simulink model "fault_tolerant_controller"  (R2015a)
settings: Solver=ode45  SolverMode=SingleTasking  StartTime=0.0  StopTime=150  RelTol=1e-3
values from neighbouring files (symbols this model uses):
  g = 9.8    [model.mat]
  Kd = 1e-06    [model.mat]
  Kt = 1    [model.mat]
  U0 = 120    [model.mat]
  X0 = 0    [model.mat]
  Y0 = 5000    [model.mat]
undefined symbols (not defined in the file or in its folder): magnitude
libraries: simulink x53, aerolibatmos2 x12, aerolibconvert2 x4
(part 1 of 2)
settings Model: CovMetricSettings=dwe  CovHtmlReporting=off  covSaveCumulativeToWorkspaceVar=off  CovSaveSingleToWorkspaceVar=off  CovExternalEMLEnable=on  Creator=jomig  LastModifiedBy=Tiago Alexandre
settings DataIOCC: LimitDataPoints=off  SaveFormat=Dataset
settings DebuggingCC: SFUnexpectedBacktrackingDiag=error  SFNoUnconditionalDefaultTransitionDiag=error
settings HardwareCC: ProdBitPerPointer=64  ProdLargestAtomicFloat=Float  ProdIntDivRoundTo=Zero  ProdEndianess=LittleEndian  ProdHWDeviceType=Specified
settings ModelReferenceCC: PropagateSignalLabelsOutOfModel=on
settings GRTTargetCC: TargetLangStandard=C99 (ISO)  GeneratePreprocessorConditionals=Use local settings

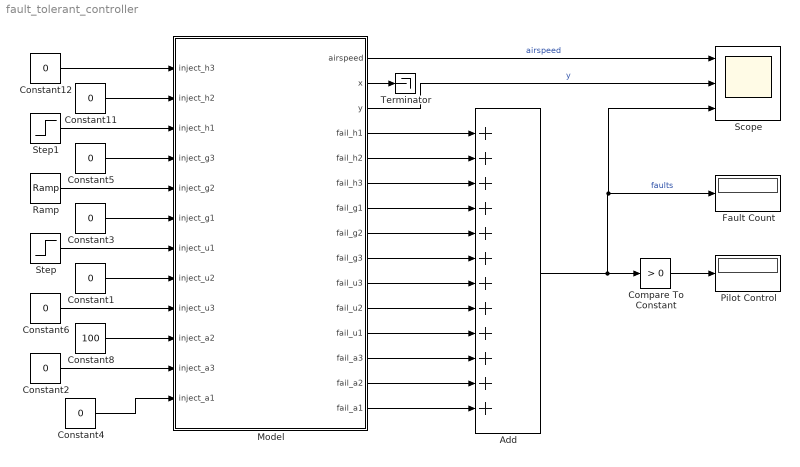
== system fault_tolerant_controller ==
  Add : Sum  Inputs=++++++++++++
  Compare To Constant : simulink/Logic and Bit Operations/Compare To Constant  relop=>  const=0  OutDataTypeStr=boolean
  Constant{1..6,11..12} (8 alike) : Constant  Value=0
  Constant8 : Constant  Value=100
  Fault Count : Display
  Model : Subsystem
  Pilot Control : Display
  Ramp : simulink/Sources/Ramp  slope=5  start=50  X0=0
  Scope : Scope  NumInputPorts=3
      settings: TimeRange=150  YMin=119~4800~1  YMax=121~5600~4
  Step : Step  Time=25  After=25  SampleTime=0
  Step1 : Step  Time=35  After=-5000  SampleTime=0
  Terminator : Terminator
  wires:
  Model/1(airspeed) -> Scope/1  "airspeed"
  Model/4(fail_h1) -> Add/1
  Model/5(fail_h2) -> Add/2
  Model/6(fail_h3) -> Add/3
  Model/7(fail_g1) -> Add/4
  Model/8(fail_g2) -> Add/5
  Model/9(fail_g3) -> Add/6
  Model/10(fail_u3) -> Add/7
  Model/11(fail_u2) -> Add/8
  Model/12(fail_u1) -> Add/9
  Model/13(fail_a3) -> Add/10
  Model/14(fail_a2) -> Add/11
  Model/15(fail_a1) -> Add/12
  Compare To Constant/1 -> Pilot Control/1
  Add/1 -> Scope/3, Fault Count/1, Compare To Constant/1  "faults"
  Constant8/1 -> Model/10(inject_a2)
  Constant6/1 -> Model/9(inject_u3)
  Constant1/1 -> Model/8(inject_u2)
  Step/1 -> Model/7(inject_u1)
  Constant3/1 -> Model/6(inject_g1)
  Ramp/1 -> Model/5(inject_g2)
  Constant5/1 -> Model/4("inject_g3 ")
  Step1/1 -> Model/3(inject_h1)
  Constant11/1 -> Model/2(inject_h2)
  Constant12/1 -> Model/1(inject_h3)
  Constant2/1 -> Model/11(inject_a3)
  Model/3(y) -> Scope/2  "y"
  Model/2(x) -> Terminator/1
  Constant4/1 -> Model/12(inject_a1)

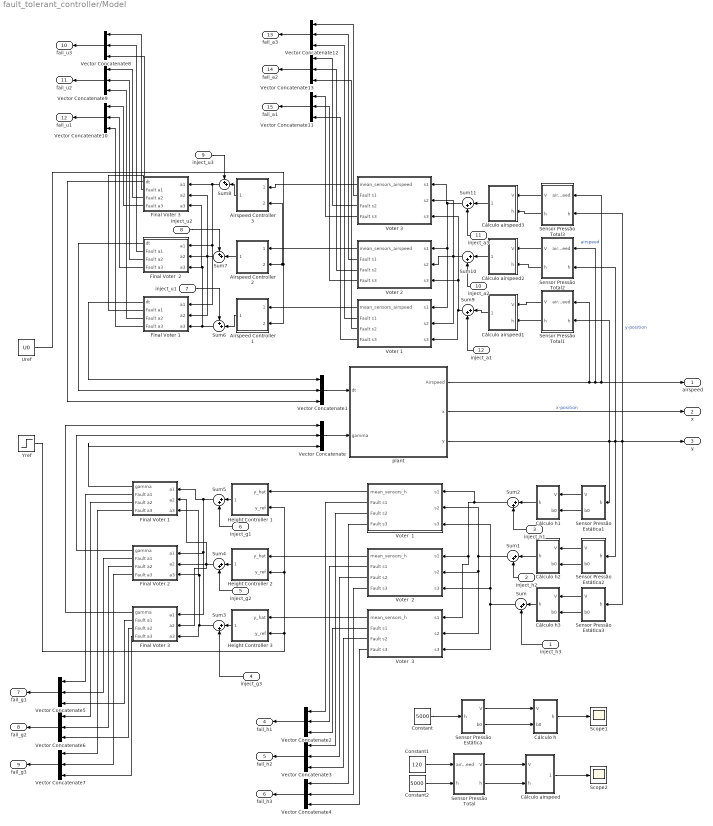
== system fault_tolerant_controller/Model ==
  inject_h3 : Inport
  inject_h2 : Inport  Port=2
  inject_h1 : Inport  Port=3
  "inject_g3 " : Inport  Port=4
  inject_g2 : Inport  Port=5
  inject_g1 : Inport  Port=6
  inject_u1 : Inport  Port=7
  inject_u2 : Inport  Port=8
  inject_u3 : Inport  Port=9
  inject_a2 : Inport  Port=10
  inject_a3 : Inport  Port=11
  inject_a1 : Inport  Port=12
  Airspeed Controller 1 : Subsystem
  Airspeed Controller 2 : Subsystem
  Airspeed Controller 3 : Subsystem
  Constant : Constant  Value=5000
  Constant1 : Constant  Value=120
  Constant2 : Constant  Value=5000
  Cálculo airspeed : Subsystem
  Cálculo airspeed1 : Subsystem
  Cálculo airspeed2 : Subsystem
  Cálculo airspeed3 : Subsystem
  Cálculo h : Subsystem
  Cálculo h1 : Subsystem
  Cálculo h2 : Subsystem
  Cálculo h3 : Subsystem
  "Final Voter  2 " : Subsystem
  Final Voter 1 : Subsystem
  "Final Voter 1   " : Subsystem
  Final Voter 2 : Subsystem
  Final Voter 3 : Subsystem
  "Final Voter 3 " : Subsystem
  Height Controller 1 : Subsystem
  Height Controller 2 : Subsystem
  Height Controller 3 : Subsystem
  Scope1 : Scope
      settings: YMin=4967.8967  YMax=5030.01388  SaveName=ScopeData5
  Scope2 : Scope
      settings: TimeRange=150  YMin=117.5  YMax=122  SaveName=ScopeData6
  Sensor Pressão Estática : Subsystem
  Sensor Pressão Estática1 : Subsystem
  Sensor Pressão Estática2 : Subsystem
  Sensor Pressão Estática3 : Subsystem
  Sensor Pressão Total : Subsystem
  Sensor Pressão Total1 : Subsystem
  Sensor Pressão Total2 : Subsystem
  Sensor Pressão Total3 : Subsystem
  Sum{,1..5,9..11} (9 alike) : Sum  Inputs=|++
  Sum6 : Sum  Inputs=++|
  Sum7 : Sum  Inputs=++|
  Sum8 : Sum  Inputs=++|
  "Uref " : Constant  Value=U0
  Vector Concatenate{,1..13} (14 alike) : Concatenate  NumInputs=3
  Voter  1 : Subsystem
  Voter  2 : Subsystem
  Voter  3 : Subsystem
  Voter 1 : Subsystem
  Voter 2 : Subsystem
  "Voter 3  " : Subsystem
  Yref : Step  Time=5  Before=Y0  After=Y0+500  SampleTime=0
  "plant " : Subsystem
  airspeed : Outport
  x : Outport  Port=2
  y : Outport  Port=3
  fail_h1 : Outport  Port=4
  fail_h2 : Outport  Port=5
  fail_h3 : Outport  Port=6
  fail_g1 : Outport  Port=7
  fail_g2 : Outport  Port=8
  fail_g3 : Outport  Port=9
  fail_u3 : Outport  Port=10
  fail_u2 : Outport  Port=11
  fail_u1 : Outport  Port=12
  fail_a3 : Outport  Port=13
  fail_a2 : Outport  Port=14
  fail_a1 : Outport  Port=15
  wires:
  "Final Voter 3 "/3(Fault a2) -> Vector Concatenate9/1
  Voter 1/3("Fault s2  ") -> Vector Concatenate13/3
  "Final Voter 1   "/4(Fault a3) -> Vector Concatenate10/3
  "Final Voter  2 "/2(Fault a1) -> Vector Concatenate8/2
  Final Voter 1/3(Fault a2) -> Vector Concatenate6/1
  Final Voter 2/2(Fault a1) -> Vector Concatenate5/2
  Final Voter 1/4(Fault a3) -> Vector Concatenate7/1
  Voter 2/4("Fault s3  ") -> Vector Concatenate11/2
  "Voter 3  "/4("Fault s3  ") -> Vector Concatenate11/1
  Final Voter 2/4(Fault a3) -> Vector Concatenate7/2
  "Final Voter  2 "/3(Fault a2) -> Vector Concatenate9/2
  Voter  2/3("Fault s2  ") -> Vector Concatenate3/2
  Final Voter 1/2(Fault a1) -> Vector Concatenate5/1
  Final Voter 3/4(Fault a3) -> Vector Concatenate7/3
  Sum/1 -> Voter  3/3(s3), Voter  2/3(s3), Voter  1/3(s3)
  Vector Concatenate5/1 -> fail_g1/1
  Vector Concatenate7/1 -> fail_g3/1
  Vector Concatenate6/1 -> fail_g2/1
  Vector Concatenate10/1 -> fail_u1/1
  Vector Concatenate8/1 -> fail_u3/1
  Vector Concatenate9/1 -> fail_u2/1
  "Voter 3  "/3("Fault s2  ") -> Vector Concatenate13/1
  Final Voter 3/3(Fault a2) -> Vector Concatenate6/3
  "Voter 3  "/2("Fault s1  ") -> Vector Concatenate12/1
  Voter 2/2("Fault s1  ") -> Vector Concatenate12/2
  Sum11/1 -> Voter 1/1(s1), Voter 2/1(s1), "Voter 3  "/1(s1)
  Height Controller 3/1(gamma) -> Sum3/1
  Airspeed Controller 2/1(Throtle) -> Sum7/2
  Sum6/1 -> "Final Voter 3 "/3(a3), "Final Voter  2 "/3(a3), "Final Voter 1   "/3(a3)
  Sum7/1 -> "Final Voter 3 "/2(a2), "Final Voter 1   "/2(a2), "Final Voter  2 "/2(a2)
  Sum8/1 -> "Final Voter 1   "/1(a1), "Final Voter  2 "/1(a1), "Final Voter 3 "/1(a1)
  Airspeed Controller 1/1(Throtle) -> Sum6/2
  Voter 2/3("Fault s2  ") -> Vector Concatenate13/2
  Voter  3/2("Fault s1  ") -> Vector Concatenate2/3
  Voter  2/2("Fault s1  ") -> Vector Concatenate2/2
  Vector Concatenate2/1 -> fail_h1/1
  Sum4/1 -> Final Voter 1/2(a2), Final Voter 3/2(a2), Final Voter 2/2(a2)
  "Final Voter 3 "/4(Fault a3) -> Vector Concatenate10/1
  Cálculo h2/1(h) -> Sum1/1
  Vector Concatenate12/1 -> fail_a3/1
  Final Voter 3/2(Fault a1) -> Vector Concatenate5/3
  Vector Concatenate11/1 -> fail_a1/1
  Vector Concatenate13/1 -> fail_a2/1
  "Final Voter  2 "/4(Fault a3) -> Vector Concatenate10/2
  Voter 1/2("Fault s1  ") -> Vector Concatenate12/3
  Voter 1/4("Fault s3  ") -> Vector Concatenate11/3
  Voter  2/4("Fault s3  ") -> Vector Concatenate4/2
  Vector Concatenate4/1 -> fail_h3/1
  inject_h3/1 -> Sum/2
  inject_h2/1 -> Sum1/2
  Voter  1/2("Fault s1  ") -> Vector Concatenate2/1
  Voter  3/3("Fault s2  ") -> Vector Concatenate3/3
  Vector Concatenate3/1 -> fail_h2/1
  "Final Voter 1   "/2(Fault a1) -> Vector Concatenate8/3
  Final Voter 2/3(Fault a2) -> Vector Concatenate6/2
  Cálculo airspeed3/1(airspeed) -> Sum11/1
  inject_u2/1 -> Sum7/1
  Voter  1/4("Fault s3  ") -> Vector Concatenate4/1
  Cálculo h3/1(h) -> Sum/1
  Airspeed Controller 3/1(Throtle) -> Sum8/2
  inject_u3/1 -> Sum8/1
  inject_u1/1 -> Sum6/1
  inject_a3/1 -> Sum11/2
  inject_a1/1 -> Sum9/2
  inject_a2/1 -> Sum10/2
  Sum9/1 -> Voter 1/3(s3), Voter 2/3(s3), "Voter 3  "/3(s3)
  Sum10/1 -> Voter 1/2(s2), Voter 2/2(s2), "Voter 3  "/2(s2)
  Cálculo airspeed1/1(airspeed) -> Sum9/1
  Voter  1/3("Fault s2  ") -> Vector Concatenate3/1
  inject_h1/1 -> Sum2/2
  Voter  3/4("Fault s3  ") -> Vector Concatenate4/3
  "Final Voter 1   "/3(Fault a2) -> Vector Concatenate9/3
  Sum2/1 -> Voter  1/1(s1), Voter  2/1(s1), Voter  3/1(s1)
  "inject_g3 "/1 -> Sum3/2
  "plant "/2(x) -> x/1  "x-position"
  "plant "/1(Airspeed) -> Sensor Pressão Total1/1(airspeed), Sensor Pressão Total2/1(airspeed), Sensor Pressão Total3/1(airspeed), airspeed/1  "airspeed"
  Sensor Pressão Estática/1(V) -> Cálculo h/1(V)
  "plant "/3(y) -> Sensor Pressão Total1/2(h), Sensor Pressão Estática1/1(h), Sensor Pressão Total2/2(h), Sensor Pressão Estática2/1(h), Sensor Pressão Total3/2(h), y/1, Sensor Pressão Estática3/1(h)  "y-position"
  Constant/1 -> Sensor Pressão Estática/1(h)
  Cálculo h/1(h) -> Scope1/1
  Voter  2/1(" mean_sensors_h") -> Height Controller 2/1(y_hat)
  Sensor Pressão Estática/2(b0) -> Cálculo h/2(b0)
  Sensor Pressão Estática3/1(V) -> Cálculo h3/1(V)
  Voter  3/1(" mean_sensors_h") -> Height Controller 3/1(y_hat)
  Sensor Pressão Estática1/1(V) -> Cálculo h1/1(V)
  Yref/1 -> Height Controller 3/2(y_ref), Height Controller 2/2(y_ref), Height Controller 1/2(y_ref)
  Voter  1/1(" mean_sensors_h") -> Height Controller 1/1(y_hat)
  Sensor Pressão Estática2/2(b0) -> Cálculo h2/2(b0)
  Sensor Pressão Estática3/2(b0) -> Cálculo h3/2(b0)
  Sensor Pressão Estática2/1(V) -> Cálculo h2/1(V)
  Sensor Pressão Estática1/2(b0) -> Cálculo h1/2(b0)
  Final Voter 1/1(gamma) -> Vector Concatenate/3
  Sensor Pressão Total3/1(V) -> Cálculo airspeed3/1("V ")
  Sensor Pressão Total1/2("h ") -> Cálculo airspeed1/2(h)
  Final Voter 2/1(gamma) -> Vector Concatenate/2
  Sensor Pressão Total3/2("h ") -> Cálculo airspeed3/2(h)
  Sensor Pressão Total2/1(V) -> Cálculo airspeed2/1("V ")
  Sensor Pressão Total2/2("h ") -> Cálculo airspeed2/2(h)
  Voter 2/1(" mean_sensors_airspeed") -> Airspeed Controller 2/1(U_hat)
  "Uref "/1 -> Airspeed Controller 1/2(U_ref), Airspeed Controller 3/2(U_ref), Airspeed Controller 2/2(U_ref)
  "Voter 3  "/1(" mean_sensors_airspeed") -> Airspeed Controller 3/1(U_hat)
  Sensor Pressão Total1/1(V) -> Cálculo airspeed1/1("V ")
  Final Voter 3/1(gamma) -> Vector Concatenate/1
  Voter 1/1(" mean_sensors_airspeed") -> Airspeed Controller 1/1(U_hat)
  Sum5/1 -> Final Voter 3/1(a1), Final Voter 2/1(a1), Final Voter 1/1(a1)
  "Final Voter 3 "/2(Fault a1) -> Vector Concatenate8/1
  Sum1/1 -> Voter  1/2(s2), Voter  2/2(s2), Voter  3/2(s2)
  "Final Voter  2 "/1(dt) -> Vector Concatenate1/2
  Vector Concatenate/1 -> "plant "/2("gamma ")
  Height Controller 1/1(gamma) -> Sum5/1
  "Final Voter 1   "/1(dt) -> Vector Concatenate1/1
  Vector Concatenate1/1 -> "plant "/1(dt)
  "Final Voter 3 "/1(dt) -> Vector Concatenate1/3
  Sum3/1 -> Final Voter 1/3(a3), Final Voter 2/3(a3), Final Voter 3/3(a3)
  inject_g2/1 -> Sum4/2
  Height Controller 2/1(gamma) -> Sum4/1
  inject_g1/1 -> Sum5/2
  Cálculo h1/1(h) -> Sum2/1
  Constant2/1 -> Sensor Pressão Total/2(h)
  Constant1/1 -> Sensor Pressão Total/1(airspeed)
  Cálculo airspeed/1(airspeed) -> Scope2/1
  Sensor Pressão Total/1(V) -> Cálculo airspeed/1("V ")
  Sensor Pressão Total/2("h ") -> Cálculo airspeed/2(h)
  Cálculo airspeed2/1(airspeed) -> Sum10/1

== system fault_tolerant_controller/Model/Airspeed Controller 1 ==
  U_hat : Inport
  U_ref : Inport  Port=2
  Integrator : Integrator
  PID Controller : simulink/Continuous/PID Controller  Controller=PID  TimeDomain=Continuous-time  SampleTime=-1  IntegratorMethod=Forward Euler  FilterMethod=Forward Euler  Form=Parallel  UseFilter=on  ControllerParametersSource=internal  P=0.3  I=0.215  D=1.1625  N=100  InitialConditionSource=internal  InitialConditionForIntegrator=0  InitialConditionForFilter=0  ExternalReset=none  LimitOutput=off  UpperSaturationLimit=inf  LowerSaturationLimit=-inf  LinearizeAsGain=on  AntiWindupMode=none  Kb=1  TrackingMode=off  Kt=1  PParamMin=[]  PParamMax=[]  IParamMin=[]  IParamMax=[]  DParamMin=[]  DParamMax=[]  NParamMin=[]  NParamMax=[]  KbParamMin=[]  KbParamMax=[]  KtParamMin=[]  KtParamMax=[]  POutMin=[]  POutMax=[]  IOutMin=[]  IOutMax=[]  DOutMin=[]  DOutMax=[]  NOutMin=[]  NOutMax=[]  KbOutMin=[]  KbOutMax=[]  KtOutMin=[]  KtOutMax=[]  IntegratorOutMin=[]  IntegratorOutMax=[]  FilterOutMin=[]  FilterOutMax=[]  SumOutMin=[]  SumOutMax=[]  SumI1OutMin=[]  SumI1OutMax=[]  SumI2OutMin=[]  SumI2OutMax=[]  SumI3OutMin=[]  SumI3OutMax=[]  SumDOutMin=[]  SumDOutMax=[]  SaturationOutMin=[]  SaturationOutMax=[]  IntegratorContinuousStateAttributes=''  IntegratorStateMustResolveToSignalObject=off  IntegratorRTWStateStorageClass=Auto  FilterContinuousStateAttributes=''  FilterStateMustResolveToSignalObject=off  FilterRTWStateStorageClass=Auto  DifferentiatorICPrevScaledInput=0  DifferentiatorOutMin=[]  DifferentiatorOutMax=[]
  Sum : Sum  Inputs=-+|
  Throtle : Outport
  wires:
  PID Controller/1 -> Integrator/1
  U_ref/1 -> Sum/2
  Integrator/1 -> Throtle/1
  U_hat/1 -> Sum/1
  Sum/1 -> PID Controller/1  "dt"

== system fault_tolerant_controller/Model/Airspeed Controller 2 ==
  U_hat : Inport
  U_ref : Inport  Port=2
  Integrator : Integrator
  PID Controller : simulink/Continuous/PID Controller  Controller=PID  TimeDomain=Continuous-time  SampleTime=-1  IntegratorMethod=Forward Euler  FilterMethod=Forward Euler  Form=Parallel  UseFilter=on  ControllerParametersSource=internal  P=0.3  I=0.215  D=1.1625  N=100  InitialConditionSource=internal  InitialConditionForIntegrator=0  InitialConditionForFilter=0  ExternalReset=none  LimitOutput=off  UpperSaturationLimit=inf  LowerSaturationLimit=-inf  LinearizeAsGain=on  AntiWindupMode=none  Kb=1  TrackingMode=off  Kt=1  PParamMin=[]  PParamMax=[]  IParamMin=[]  IParamMax=[]  DParamMin=[]  DParamMax=[]  NParamMin=[]  NParamMax=[]  KbParamMin=[]  KbParamMax=[]  KtParamMin=[]  KtParamMax=[]  POutMin=[]  POutMax=[]  IOutMin=[]  IOutMax=[]  DOutMin=[]  DOutMax=[]  NOutMin=[]  NOutMax=[]  KbOutMin=[]  KbOutMax=[]  KtOutMin=[]  KtOutMax=[]  IntegratorOutMin=[]  IntegratorOutMax=[]  FilterOutMin=[]  FilterOutMax=[]  SumOutMin=[]  SumOutMax=[]  SumI1OutMin=[]  SumI1OutMax=[]  SumI2OutMin=[]  SumI2OutMax=[]  SumI3OutMin=[]  SumI3OutMax=[]  SumDOutMin=[]  SumDOutMax=[]  SaturationOutMin=[]  SaturationOutMax=[]  IntegratorContinuousStateAttributes=''  IntegratorStateMustResolveToSignalObject=off  IntegratorRTWStateStorageClass=Auto  FilterContinuousStateAttributes=''  FilterStateMustResolveToSignalObject=off  FilterRTWStateStorageClass=Auto  DifferentiatorICPrevScaledInput=0  DifferentiatorOutMin=[]  DifferentiatorOutMax=[]
  Sum : Sum  Inputs=-+|
  Throtle : Outport
  wires:
  PID Controller/1 -> Integrator/1
  U_ref/1 -> Sum/2
  Integrator/1 -> Throtle/1
  U_hat/1 -> Sum/1
  Sum/1 -> PID Controller/1  "dt"

== system fault_tolerant_controller/Model/Airspeed Controller 3 ==
  U_hat : Inport
  U_ref : Inport  Port=2
  Integrator : Integrator
  PID Controller : simulink/Continuous/PID Controller  Controller=PID  TimeDomain=Continuous-time  SampleTime=-1  IntegratorMethod=Forward Euler  FilterMethod=Forward Euler  Form=Parallel  UseFilter=on  ControllerParametersSource=internal  P=0.3  I=0.215  D=1.1625  N=100  InitialConditionSource=internal  InitialConditionForIntegrator=0  InitialConditionForFilter=0  ExternalReset=none  LimitOutput=off  UpperSaturationLimit=inf  LowerSaturationLimit=-inf  LinearizeAsGain=on  AntiWindupMode=none  Kb=1  TrackingMode=off  Kt=1  PParamMin=[]  PParamMax=[]  IParamMin=[]  IParamMax=[]  DParamMin=[]  DParamMax=[]  NParamMin=[]  NParamMax=[]  KbParamMin=[]  KbParamMax=[]  KtParamMin=[]  KtParamMax=[]  POutMin=[]  POutMax=[]  IOutMin=[]  IOutMax=[]  DOutMin=[]  DOutMax=[]  NOutMin=[]  NOutMax=[]  KbOutMin=[]  KbOutMax=[]  KtOutMin=[]  KtOutMax=[]  IntegratorOutMin=[]  IntegratorOutMax=[]  FilterOutMin=[]  FilterOutMax=[]  SumOutMin=[]  SumOutMax=[]  SumI1OutMin=[]  SumI1OutMax=[]  SumI2OutMin=[]  SumI2OutMax=[]  SumI3OutMin=[]  SumI3OutMax=[]  SumDOutMin=[]  SumDOutMax=[]  SaturationOutMin=[]  SaturationOutMax=[]  IntegratorContinuousStateAttributes=''  IntegratorStateMustResolveToSignalObject=off  IntegratorRTWStateStorageClass=Auto  FilterContinuousStateAttributes=''  FilterStateMustResolveToSignalObject=off  FilterRTWStateStorageClass=Auto  DifferentiatorICPrevScaledInput=0  DifferentiatorOutMin=[]  DifferentiatorOutMax=[]
  Sum : Sum  Inputs=-+|
  Throtle : Outport
  wires:
  PID Controller/1 -> Integrator/1
  U_ref/1 -> Sum/2
  Integrator/1 -> Throtle/1
  U_hat/1 -> Sum/1
  Sum/1 -> PID Controller/1  "dt"

== system fault_tolerant_controller/Model/Cálculo airspeed ==
  "V " : Inport
  h : Inport  Port=2
  Constant1 : Constant  Value=2
  Divide : Product  Inputs=*/
  ISA Atmosphere Model : aerolibatmos2/ISA Atmosphere Model  custom=on  g=9.80665  gamma=1.4  R=287.0531  L=0.0065  h_trop=11000  h_strat=20000  rho0=1.225  P0=101325  T0=288.15  h0=0
  Pressão Dinâmica : Sum  Inputs=+-
  Pressão Total : Fcn  Expr=u*(165125/5)
  Product : Product
  Sqrt : Sqrt  SaturateOnIntegerOverflow=on
  airspeed : Outport
  wires:
  "V "/1 -> Pressão Total/1
  Divide/1 -> Sqrt/1
  Product/1 -> Divide/1
  Sqrt/1 -> airspeed/1
  Constant1/1 -> Product/2
  Pressão Total/1 -> Pressão Dinâmica/1
  Pressão Dinâmica/1 -> Product/1
  h/1 -> ISA Atmosphere Model/1
  ISA Atmosphere Model/3 -> Pressão Dinâmica/2
  ISA Atmosphere Model/4 -> Divide/2

== system fault_tolerant_controller/Model/Cálculo airspeed1 ==
  "V " : Inport
  h : Inport  Port=2
  Constant1 : Constant  Value=2
  Divide : Product  Inputs=*/
  ISA Atmosphere Model : aerolibatmos2/ISA Atmosphere Model  custom=on  g=9.80665  gamma=1.4  R=287.0531  L=0.0065  h_trop=11000  h_strat=20000  rho0=1.225  P0=101325  T0=288.15  h0=0
  Pressão Dinâmica : Sum  Inputs=+-
  Pressão Total : Fcn  Expr=u*(165125/5)
  Product : Product
  Sqrt : Sqrt  SaturateOnIntegerOverflow=on
  airspeed : Outport
  wires:
  "V "/1 -> Pressão Total/1
  Divide/1 -> Sqrt/1
  Product/1 -> Divide/1
  Sqrt/1 -> airspeed/1
  Constant1/1 -> Product/2
  Pressão Total/1 -> Pressão Dinâmica/1
  Pressão Dinâmica/1 -> Product/1
  h/1 -> ISA Atmosphere Model/1
  ISA Atmosphere Model/3 -> Pressão Dinâmica/2
  ISA Atmosphere Model/4 -> Divide/2

== system fault_tolerant_controller/Model/Cálculo airspeed2 ==
  "V " : Inport
  h : Inport  Port=2
  Constant1 : Constant  Value=2
  Divide : Product  Inputs=*/
  ISA Atmosphere Model : aerolibatmos2/ISA Atmosphere Model  custom=on  g=9.80665  gamma=1.4  R=287.0531  L=0.0065  h_trop=11000  h_strat=20000  rho0=1.225  P0=101325  T0=288.15  h0=0
  Pressão Dinâmica : Sum  Inputs=+-
  Pressão Total : Fcn  Expr=u*(165125/5)
  Product : Product
  Sqrt : Sqrt  SaturateOnIntegerOverflow=on
  airspeed : Outport
  wires:
  "V "/1 -> Pressão Total/1
  Divide/1 -> Sqrt/1
  Product/1 -> Divide/1
  Sqrt/1 -> airspeed/1
  Constant1/1 -> Product/2
  Pressão Total/1 -> Pressão Dinâmica/1
  Pressão Dinâmica/1 -> Product/1
  h/1 -> ISA Atmosphere Model/1
  ISA Atmosphere Model/3 -> Pressão Dinâmica/2
  ISA Atmosphere Model/4 -> Divide/2

== system fault_tolerant_controller/Model/Cálculo airspeed3 ==
  "V " : Inport
  h : Inport  Port=2
  Constant1 : Constant  Value=2
  Divide : Product  Inputs=*/
  ISA Atmosphere Model : aerolibatmos2/ISA Atmosphere Model  custom=on  g=9.80665  gamma=1.4  R=287.0531  L=0.0065  h_trop=11000  h_strat=20000  rho0=1.225  P0=101325  T0=288.15  h0=0
  Pressão Dinâmica : Sum  Inputs=+-
  Pressão Total : Fcn  Expr=u*(165125/5)
  Product : Product
  Sqrt : Sqrt  SaturateOnIntegerOverflow=on
  airspeed : Outport
  wires:
  "V "/1 -> Pressão Total/1
  Divide/1 -> Sqrt/1
  Product/1 -> Divide/1
  Sqrt/1 -> airspeed/1
  Constant1/1 -> Product/2
  Pressão Total/1 -> Pressão Dinâmica/1
  Pressão Dinâmica/1 -> Product/1
  h/1 -> ISA Atmosphere Model/1
  ISA Atmosphere Model/3 -> Pressão Dinâmica/2
  ISA Atmosphere Model/4 -> Divide/2

== system fault_tolerant_controller/Model/Cálculo h ==
  V : Inport
  b0 : Inport  Port=2
  Modelo ISA : Fcn  Expr=(1-(u/101325)^(1/5.25588))*(288.15/0.0065)
  Subtract : Sum  Inputs=-+
  p : Fcn  Expr=(-0.0023+sqrt(0.0023^2-4*1.926e-6*u))/(2*1.926e-6)
  h : Outport
  wires:
  Subtract/1 -> p/1
  b0/1 -> Subtract/2
  V/1 -> Subtract/1
  p/1 -> Modelo ISA/1
  Modelo ISA/1 -> h/1

== system fault_tolerant_controller/Model/Cálculo h1 ==
  V : Inport
  b0 : Inport  Port=2
  Modelo ISA : Fcn  Expr=(1-(u/101325)^(1/5.25588))*(288.15/0.0065)
  Subtract : Sum  Inputs=-+
  p : Fcn  Expr=(-0.0023+sqrt(0.0023^2-4*1.926e-6*u))/(2*1.926e-6)
  h : Outport
  wires:
  Subtract/1 -> p/1
  b0/1 -> Subtract/2
  V/1 -> Subtract/1
  p/1 -> Modelo ISA/1
  Modelo ISA/1 -> h/1

== system fault_tolerant_controller/Model/Cálculo h2 ==
  V : Inport
  b0 : Inport  Port=2
  Modelo ISA : Fcn  Expr=(1-(u/101325)^(1/5.25588))*(288.15/0.0065)
  Subtract : Sum  Inputs=-+
  p : Fcn  Expr=(-0.0023+sqrt(0.0023^2-4*1.926e-6*u))/(2*1.926e-6)
  h : Outport
  wires:
  Subtract/1 -> p/1
  b0/1 -> Subtract/2
  V/1 -> Subtract/1
  p/1 -> Modelo ISA/1
  Modelo ISA/1 -> h/1

== system fault_tolerant_controller/Model/Cálculo h3 ==
  V : Inport
  b0 : Inport  Port=2
  Modelo ISA : Fcn  Expr=(1-(u/101325)^(1/5.25588))*(288.15/0.0065)
  Subtract : Sum  Inputs=-+
  p : Fcn  Expr=(-0.0023+sqrt(0.0023^2-4*1.926e-6*u))/(2*1.926e-6)
  h : Outport
  wires:
  Subtract/1 -> p/1
  b0/1 -> Subtract/2
  V/1 -> Subtract/1
  p/1 -> Modelo ISA/1
  Modelo ISA/1 -> h/1

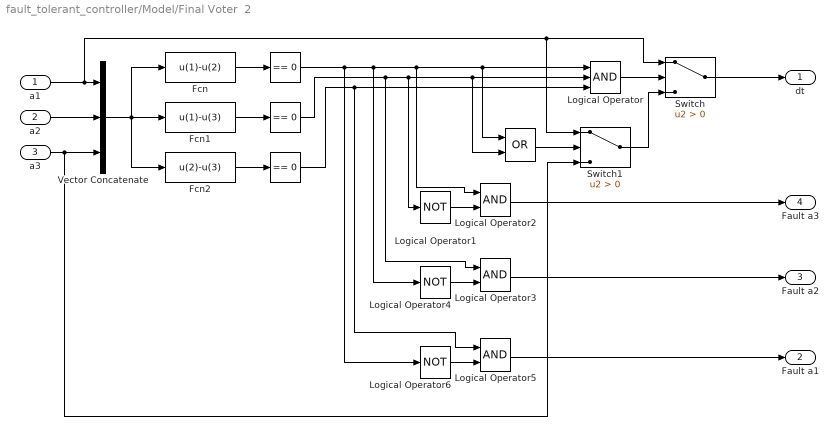
== system fault_tolerant_controller/Model/Final Voter  2  ==
  a1 : Inport
  a2 : Inport  Port=2
  a3 : Inport  Port=3
  " " : simulink/Logic and Bit Operations/Compare To Zero  relop===  OutDataTypeStr=boolean
  "  " : Logic  Operator=OR  AllPortsSameDT=off  OutDataTypeStr=boolean
  "   " : simulink/Logic and Bit Operations/Compare To Zero  relop===  OutDataTypeStr=boolean
  "                                   " : simulink/Logic and Bit Operations/Compare To Zero  relop===  OutDataTypeStr=boolean
  Fcn : Fcn  Expr=u(1)-u(2)
  Fcn1 : Fcn  Expr=u(1)-u(3)
  Fcn2 : Fcn  Expr=u(2)-u(3)
  Logical Operator : Logic  Inputs=3  AllPortsSameDT=off  OutDataTypeStr=boolean
  Logical Operator1 : Logic  Operator=NOT  AllPortsSameDT=off  OutDataTypeStr=boolean
  Logical Operator2 : Logic  AllPortsSameDT=off  OutDataTypeStr=boolean
  Logical Operator3 : Logic  AllPortsSameDT=off  OutDataTypeStr=boolean
  Logical Operator4 : Logic  Operator=NOT  AllPortsSameDT=off  OutDataTypeStr=boolean
  Logical Operator5 : Logic  AllPortsSameDT=off  OutDataTypeStr=boolean
  Logical Operator6 : Logic  Operator=NOT  AllPortsSameDT=off  OutDataTypeStr=boolean
  Switch : Switch  Criteria=u2 > Threshold
  Switch1 : Switch  Criteria=u2 > Threshold
  Vector Concatenate : Concatenate  NumInputs=3
  dt : Outport
  Fault a1 : Outport  Port=2
  Fault a2 : Outport  Port=3
  Fault a3 : Outport  Port=4
  wires:
  a3/1 -> Vector Concatenate/3, Switch1/3
  Vector Concatenate/1 -> Fcn2/1, Fcn1/1, Fcn/1
  a1/1 -> Switch1/1, Switch/1, Vector Concatenate/1
  a2/1 -> Vector Concatenate/2
  Fcn/1 -> " "/1
  Fcn1/1 -> "   "/1
  Fcn2/1 -> "                                   "/1
  " "/1 -> "  "/1, Logical Operator/1, Logical Operator2/1, Logical Operator4/1, Logical Operator6/1
  "   "/1 -> "  "/2, Logical Operator/2, Logical Operator1/1, Logical Operator3/1
  "                                   "/1 -> Logical Operator/3, Logical Operator5/1
  Logical Operator/1 -> Switch/2
  Switch/1 -> dt/1
  Logical Operator1/1 -> Logical Operator2/2
  Logical Operator4/1 -> Logical Operator3/2
  Logical Operator3/1 -> Fault a2/1
  Logical Operator2/1 -> Fault a3/1
  Logical Operator5/1 -> Fault a1/1
  Logical Operator6/1 -> Logical Operator5/2
  Switch1/1 -> Switch/3
  "  "/1 -> Switch1/2

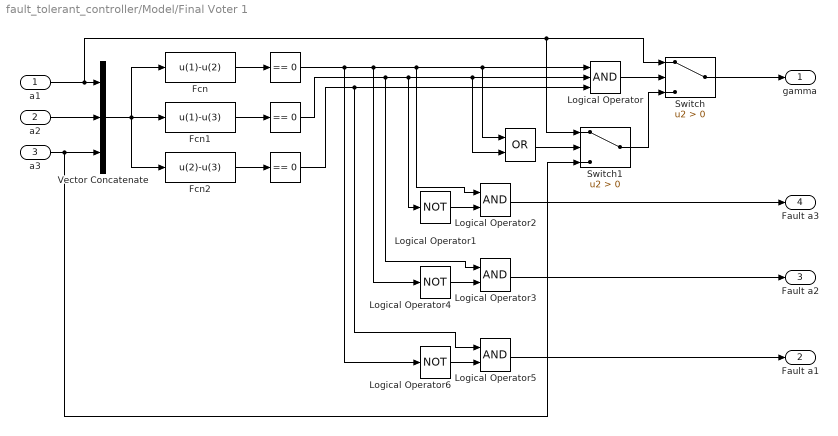
== system fault_tolerant_controller/Model/Final Voter 1 ==
  a1 : Inport
  a2 : Inport  Port=2
  a3 : Inport  Port=3
  " " : simulink/Logic and Bit Operations/Compare To Zero  relop===  OutDataTypeStr=boolean
  "  " : Logic  Operator=OR  AllPortsSameDT=off  OutDataTypeStr=boolean
  "   " : simulink/Logic and Bit Operations/Compare To Zero  relop===  OutDataTypeStr=boolean
  "                                   " : simulink/Logic and Bit Operations/Compare To Zero  relop===  OutDataTypeStr=boolean
  Fcn : Fcn  Expr=u(1)-u(2)
  Fcn1 : Fcn  Expr=u(1)-u(3)
  Fcn2 : Fcn  Expr=u(2)-u(3)
  Logical Operator : Logic  Inputs=3  AllPortsSameDT=off  OutDataTypeStr=boolean
  Logical Operator1 : Logic  Operator=NOT  AllPortsSameDT=off  OutDataTypeStr=boolean
  Logical Operator2 : Logic  AllPortsSameDT=off  OutDataTypeStr=boolean
  Logical Operator3 : Logic  AllPortsSameDT=off  OutDataTypeStr=boolean
  Logical Operator4 : Logic  Operator=NOT  AllPortsSameDT=off  OutDataTypeStr=boolean
  Logical Operator5 : Logic  AllPortsSameDT=off  OutDataTypeStr=boolean
  Logical Operator6 : Logic  Operator=NOT  AllPortsSameDT=off  OutDataTypeStr=boolean
  Switch : Switch  Criteria=u2 > Threshold
  Switch1 : Switch  Criteria=u2 > Threshold
  Vector Concatenate : Concatenate  NumInputs=3
  gamma : Outport
  Fault a1 : Outport  Port=2
  Fault a2 : Outport  Port=3
  Fault a3 : Outport  Port=4
  wires:
  a3/1 -> Vector Concatenate/3, Switch1/3
  Vector Concatenate/1 -> Fcn2/1, Fcn1/1, Fcn/1
  a1/1 -> Switch1/1, Switch/1, Vector Concatenate/1
  a2/1 -> Vector Concatenate/2
  Fcn/1 -> " "/1
  Fcn1/1 -> "   "/1
  Fcn2/1 -> "                                   "/1
  " "/1 -> "  "/1, Logical Operator/1, Logical Operator2/1, Logical Operator4/1, Logical Operator6/1
  "   "/1 -> "  "/2, Logical Operator/2, Logical Operator1/1, Logical Operator3/1
  "                                   "/1 -> Logical Operator/3, Logical Operator5/1
  Logical Operator/1 -> Switch/2
  Switch/1 -> gamma/1
  Logical Operator1/1 -> Logical Operator2/2
  Logical Operator4/1 -> Logical Operator3/2
  Logical Operator3/1 -> Fault a2/1
  Logical Operator2/1 -> Fault a3/1
  Logical Operator5/1 -> Fault a1/1
  Logical Operator6/1 -> Logical Operator5/2
  Switch1/1 -> Switch/3
  "  "/1 -> Switch1/2

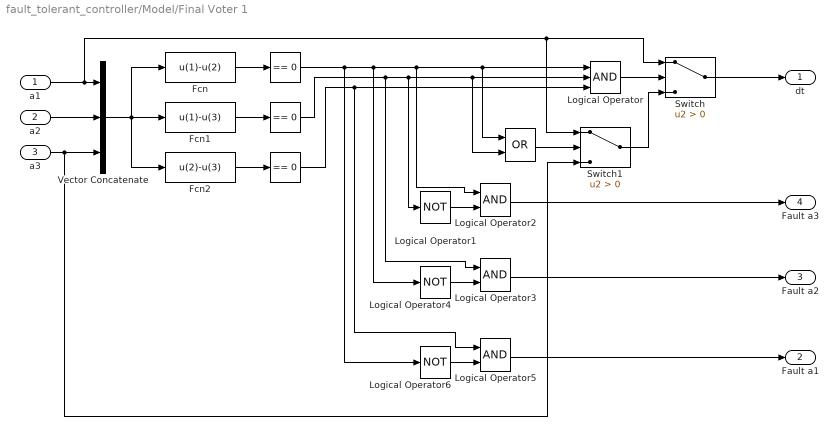
== system fault_tolerant_controller/Model/Final Voter 1    ==
  a1 : Inport
  a2 : Inport  Port=2
  a3 : Inport  Port=3
  " " : simulink/Logic and Bit Operations/Compare To Zero  relop===  OutDataTypeStr=boolean
  "  " : Logic  Operator=OR  AllPortsSameDT=off  OutDataTypeStr=boolean
  "   " : simulink/Logic and Bit Operations/Compare To Zero  relop===  OutDataTypeStr=boolean
  "                                   " : simulink/Logic and Bit Operations/Compare To Zero  relop===  OutDataTypeStr=boolean
  Fcn : Fcn  Expr=u(1)-u(2)
  Fcn1 : Fcn  Expr=u(1)-u(3)
  Fcn2 : Fcn  Expr=u(2)-u(3)
  Logical Operator : Logic  Inputs=3  AllPortsSameDT=off  OutDataTypeStr=boolean
  Logical Operator1 : Logic  Operator=NOT  AllPortsSameDT=off  OutDataTypeStr=boolean
  Logical Operator2 : Logic  AllPortsSameDT=off  OutDataTypeStr=boolean
  Logical Operator3 : Logic  AllPortsSameDT=off  OutDataTypeStr=boolean
  Logical Operator4 : Logic  Operator=NOT  AllPortsSameDT=off  OutDataTypeStr=boolean
  Logical Operator5 : Logic  AllPortsSameDT=off  OutDataTypeStr=boolean
  Logical Operator6 : Logic  Operator=NOT  AllPortsSameDT=off  OutDataTypeStr=boolean
  Switch : Switch  Criteria=u2 > Threshold
  Switch1 : Switch  Criteria=u2 > Threshold
  Vector Concatenate : Concatenate  NumInputs=3
  dt : Outport
  Fault a1 : Outport  Port=2
  Fault a2 : Outport  Port=3
  Fault a3 : Outport  Port=4
  wires:
  a3/1 -> Vector Concatenate/3, Switch1/3
  Vector Concatenate/1 -> Fcn2/1, Fcn1/1, Fcn/1
  a1/1 -> Switch1/1, Switch/1, Vector Concatenate/1
  a2/1 -> Vector Concatenate/2
  Fcn/1 -> " "/1
  Fcn1/1 -> "   "/1
  Fcn2/1 -> "                                   "/1
  " "/1 -> "  "/1, Logical Operator/1, Logical Operator2/1, Logical Operator4/1, Logical Operator6/1
  "   "/1 -> "  "/2, Logical Operator/2, Logical Operator1/1, Logical Operator3/1
  "                                   "/1 -> Logical Operator/3, Logical Operator5/1
  Logical Operator/1 -> Switch/2
  Switch/1 -> dt/1
  Logical Operator1/1 -> Logical Operator2/2
  Logical Operator4/1 -> Logical Operator3/2
  Logical Operator3/1 -> Fault a2/1
  Logical Operator2/1 -> Fault a3/1
  Logical Operator5/1 -> Fault a1/1
  Logical Operator6/1 -> Logical Operator5/2
  Switch1/1 -> Switch/3
  "  "/1 -> Switch1/2

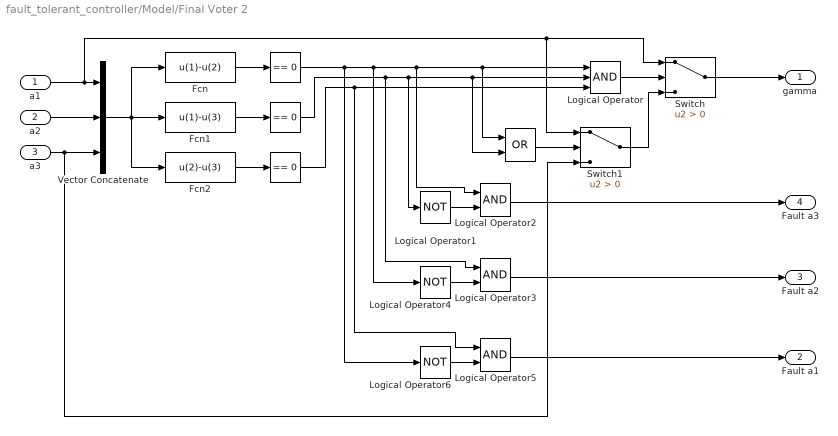
== system fault_tolerant_controller/Model/Final Voter 2 ==
  a1 : Inport
  a2 : Inport  Port=2
  a3 : Inport  Port=3
  " " : simulink/Logic and Bit Operations/Compare To Zero  relop===  OutDataTypeStr=boolean
  "  " : Logic  Operator=OR  AllPortsSameDT=off  OutDataTypeStr=boolean
  "   " : simulink/Logic and Bit Operations/Compare To Zero  relop===  OutDataTypeStr=boolean
  "                                   " : simulink/Logic and Bit Operations/Compare To Zero  relop===  OutDataTypeStr=boolean
  Fcn : Fcn  Expr=u(1)-u(2)
  Fcn1 : Fcn  Expr=u(1)-u(3)
  Fcn2 : Fcn  Expr=u(2)-u(3)
  Logical Operator : Logic  Inputs=3  AllPortsSameDT=off  OutDataTypeStr=boolean
  Logical Operator1 : Logic  Operator=NOT  AllPortsSameDT=off  OutDataTypeStr=boolean
  Logical Operator2 : Logic  AllPortsSameDT=off  OutDataTypeStr=boolean
  Logical Operator3 : Logic  AllPortsSameDT=off  OutDataTypeStr=boolean
  Logical Operator4 : Logic  Operator=NOT  AllPortsSameDT=off  OutDataTypeStr=boolean
  Logical Operator5 : Logic  AllPortsSameDT=off  OutDataTypeStr=boolean
  Logical Operator6 : Logic  Operator=NOT  AllPortsSameDT=off  OutDataTypeStr=boolean
  Switch : Switch  Criteria=u2 > Threshold
  Switch1 : Switch  Criteria=u2 > Threshold
  Vector Concatenate : Concatenate  NumInputs=3
  gamma : Outport
  Fault a1 : Outport  Port=2
  Fault a2 : Outport  Port=3
  Fault a3 : Outport  Port=4
  wires:
  a3/1 -> Vector Concatenate/3, Switch1/3
  Vector Concatenate/1 -> Fcn2/1, Fcn1/1, Fcn/1
  a1/1 -> Switch1/1, Switch/1, Vector Concatenate/1
  a2/1 -> Vector Concatenate/2
  Fcn/1 -> " "/1
  Fcn1/1 -> "   "/1
  Fcn2/1 -> "                                   "/1
  " "/1 -> "  "/1, Logical Operator/1, Logical Operator2/1, Logical Operator4/1, Logical Operator6/1
  "   "/1 -> "  "/2, Logical Operator/2, Logical Operator1/1, Logical Operator3/1
  "                                   "/1 -> Logical Operator/3, Logical Operator5/1
  Logical Operator/1 -> Switch/2
  Switch/1 -> gamma/1
  Logical Operator1/1 -> Logical Operator2/2
  Logical Operator4/1 -> Logical Operator3/2
  Logical Operator3/1 -> Fault a2/1
  Logical Operator2/1 -> Fault a3/1
  Logical Operator5/1 -> Fault a1/1
  Logical Operator6/1 -> Logical Operator5/2
  Switch1/1 -> Switch/3
  "  "/1 -> Switch1/2

== system fault_tolerant_controller/Model/Final Voter 3 ==
  a1 : Inport
  a2 : Inport  Port=2
  a3 : Inport  Port=3
  " " : simulink/Logic and Bit Operations/Compare To Zero  relop===  OutDataTypeStr=boolean
  "  " : Logic  Operator=OR  AllPortsSameDT=off  OutDataTypeStr=boolean
  "   " : simulink/Logic and Bit Operations/Compare To Zero  relop===  OutDataTypeStr=boolean
  "                                   " : simulink/Logic and Bit Operations/Compare To Zero  relop===  OutDataTypeStr=boolean
  Fcn : Fcn  Expr=u(1)-u(2)
  Fcn1 : Fcn  Expr=u(1)-u(3)
  Fcn2 : Fcn  Expr=u(2)-u(3)
  Logical Operator : Logic  Inputs=3  AllPortsSameDT=off  OutDataTypeStr=boolean
  Logical Operator1 : Logic  Operator=NOT  AllPortsSameDT=off  OutDataTypeStr=boolean
  Logical Operator2 : Logic  AllPortsSameDT=off  OutDataTypeStr=boolean
  Logical Operator3 : Logic  AllPortsSameDT=off  OutDataTypeStr=boolean
  Logical Operator4 : Logic  Operator=NOT  AllPortsSameDT=off  OutDataTypeStr=boolean
  Logical Operator5 : Logic  AllPortsSameDT=off  OutDataTypeStr=boolean
  Logical Operator6 : Logic  Operator=NOT  AllPortsSameDT=off  OutDataTypeStr=boolean
  Switch : Switch  Criteria=u2 > Threshold
  Switch1 : Switch  Criteria=u2 > Threshold
  Vector Concatenate : Concatenate  NumInputs=3
  gamma : Outport
  Fault a1 : Outport  Port=2
  Fault a2 : Outport  Port=3
  Fault a3 : Outport  Port=4
  wires:
  a3/1 -> Vector Concatenate/3, Switch1/3
  Vector Concatenate/1 -> Fcn2/1, Fcn1/1, Fcn/1
  a1/1 -> Switch1/1, Switch/1, Vector Concatenate/1
  a2/1 -> Vector Concatenate/2
  Fcn/1 -> " "/1
  Fcn1/1 -> "   "/1
  Fcn2/1 -> "                                   "/1
  " "/1 -> "  "/1, Logical Operator/1, Logical Operator2/1, Logical Operator4/1, Logical Operator6/1
  "   "/1 -> "  "/2, Logical Operator/2, Logical Operator1/1, Logical Operator3/1
  "                                   "/1 -> Logical Operator/3, Logical Operator5/1
  Logical Operator/1 -> Switch/2
  Switch/1 -> gamma/1
  Logical Operator1/1 -> Logical Operator2/2
  Logical Operator4/1 -> Logical Operator3/2
  Logical Operator3/1 -> Fault a2/1
  Logical Operator2/1 -> Fault a3/1
  Logical Operator5/1 -> Fault a1/1
  Logical Operator6/1 -> Logical Operator5/2
  Switch1/1 -> Switch/3
  "  "/1 -> Switch1/2

== system fault_tolerant_controller/Model/Final Voter 3  ==
  a1 : Inport
  a2 : Inport  Port=2
  a3 : Inport  Port=3
  " " : simulink/Logic and Bit Operations/Compare To Zero  relop===  OutDataTypeStr=boolean
  "  " : Logic  Operator=OR  AllPortsSameDT=off  OutDataTypeStr=boolean
  "   " : simulink/Logic and Bit Operations/Compare To Zero  relop===  OutDataTypeStr=boolean
  "                                   " : simulink/Logic and Bit Operations/Compare To Zero  relop===  OutDataTypeStr=boolean
  Fcn : Fcn  Expr=u(1)-u(2)
  Fcn1 : Fcn  Expr=u(1)-u(3)
  Fcn2 : Fcn  Expr=u(2)-u(3)
  Logical Operator : Logic  Inputs=3  AllPortsSameDT=off  OutDataTypeStr=boolean
  Logical Operator1 : Logic  Operator=NOT  AllPortsSameDT=off  OutDataTypeStr=boolean
  Logical Operator2 : Logic  AllPortsSameDT=off  OutDataTypeStr=boolean
  Logical Operator3 : Logic  AllPortsSameDT=off  OutDataTypeStr=boolean
  Logical Operator4 : Logic  Operator=NOT  AllPortsSameDT=off  OutDataTypeStr=boolean
  Logical Operator5 : Logic  AllPortsSameDT=off  OutDataTypeStr=boolean
  Logical Operator6 : Logic  Operator=NOT  AllPortsSameDT=off  OutDataTypeStr=boolean
  Switch : Switch  Criteria=u2 > Threshold
  Switch1 : Switch  Criteria=u2 > Threshold
  Vector Concatenate : Concatenate  NumInputs=3
  dt : Outport
  Fault a1 : Outport  Port=2
  Fault a2 : Outport  Port=3
  Fault a3 : Outport  Port=4
  wires:
  a3/1 -> Vector Concatenate/3, Switch1/3
  Vector Concatenate/1 -> Fcn2/1, Fcn1/1, Fcn/1
  a1/1 -> Switch1/1, Switch/1, Vector Concatenate/1
  a2/1 -> Vector Concatenate/2
  Fcn/1 -> " "/1
  Fcn1/1 -> "   "/1
  Fcn2/1 -> "                                   "/1
  " "/1 -> "  "/1, Logical Operator/1, Logical Operator2/1, Logical Operator4/1, Logical Operator6/1
  "   "/1 -> "  "/2, Logical Operator/2, Logical Operator1/1, Logical Operator3/1
  "                                   "/1 -> Logical Operator/3, Logical Operator5/1
  Logical Operator/1 -> Switch/2
  Switch/1 -> dt/1
  Logical Operator1/1 -> Logical Operator2/2
  Logical Operator4/1 -> Logical Operator3/2
  Logical Operator3/1 -> Fault a2/1
  Logical Operator2/1 -> Fault a3/1
  Logical Operator5/1 -> Fault a1/1
  Logical Operator6/1 -> Logical Operator5/2
  Switch1/1 -> Switch/3
  "  "/1 -> Switch1/2

== system fault_tolerant_controller/Model/Height Controller 1 ==
  y_hat : Inport
  y_ref : Inport  Port=2
  K : Gain  Gain=0.001
  Saturation : Saturate  UpperLimit=3*pi/180  LowerLimit=-3*pi/180
  Sum : Sum  Inputs=|+-
  gamma : Outport
  wires:
  Saturation/1 -> gamma/1
  y_ref/1 -> Sum/1
  y_hat/1 -> Sum/2
  K/1 -> Saturation/1
  Sum/1 -> K/1

== system fault_tolerant_controller/Model/Height Controller 2 ==
  y_hat : Inport
  y_ref : Inport  Port=2
  K : Gain  Gain=0.001
  Saturation : Saturate  UpperLimit=3*pi/180  LowerLimit=-3*pi/180
  Sum : Sum  Inputs=|+-
  gamma : Outport
  wires:
  Saturation/1 -> gamma/1
  y_ref/1 -> Sum/1
  y_hat/1 -> Sum/2
  K/1 -> Saturation/1
  Sum/1 -> K/1

== system fault_tolerant_controller/Model/Height Controller 3 ==
  y_hat : Inport
  y_ref : Inport  Port=2
  K : Gain  Gain=0.001
  Saturation : Saturate  UpperLimit=3*pi/180  LowerLimit=-3*pi/180
  Sum : Sum  Inputs=|+-
  gamma : Outport
  wires:
  Saturation/1 -> gamma/1
  y_ref/1 -> Sum/1
  y_hat/1 -> Sum/2
  K/1 -> Saturation/1
  Sum/1 -> K/1

== system fault_tolerant_controller/Model/Sensor Pressão Estática ==
  h : Inport
  "  " : Sum
  Band-Limited White Noise : simulink/Sources/Band-Limited White Noise  Cov=[10]  Ts=0.1  seed=[23341]
  Band-Limited White Noise1 : simulink/Sources/Band-Limited White Noise  Cov=[0.001]  Ts=0.1  seed=[56129]
  Conversor A/D : Quantizer  QuantizationInterval=7.629e-5
  Conversor A/D1 : Quantizer  QuantizationInterval=0.00244
  ISA Atmosphere Model : aerolibatmos2/ISA Atmosphere Model  custom=on  g=9.80665  gamma=1.4  R=287.0531  L=0.0065  h_trop=11000  h_strat=20000  rho0=1.225  P0=101325  T0=288.15  h0=0
  Product : Product
  "Product  " : Product  Inputs=3
  Sum : Sum  Inputs=|++
  Temperature Conversion : aerolibconvert2/Temperature Conversion  IU=K  OU=C
  Voltage : Sum  Inputs=+++
  "b0 " : Fcn  Expr=(4.227e-1+1.513e-2*u)/(8.615e1+u)
  b1 : Constant  Value=0.0023
  "b2 " : Constant  Value=1.926e-6
  V : Outport
  b0 : Outport  Port=2
  wires:
  b1/1 -> Product/2
  h/1 -> ISA Atmosphere Model/1
  "b0 "/1 -> b0/1, Voltage/1
  Product/1 -> Voltage/2
  ISA Atmosphere Model/1 -> Temperature Conversion/1
  ISA Atmosphere Model/3 -> "Product  "/2, "Product  "/1, Product/1
  "Product  "/1 -> Voltage/3
  Voltage/1 -> Sum/1
  "b2 "/1 -> "Product  "/3
  Band-Limited White Noise/1 -> Sum/2
  Sum/1 -> Conversor A/D/1
  Conversor A/D/1 -> V/1
  Temperature Conversion/1 -> "  "/2
  "  "/1 -> Conversor A/D1/1
  Conversor A/D1/1 -> "b0 "/1
  Band-Limited White Noise1/1 -> "  "/1

== system fault_tolerant_controller/Model/Sensor Pressão Estática1 ==
  h : Inport
  "  " : Sum
  Band-Limited White Noise : simulink/Sources/Band-Limited White Noise  Cov=[25]  Ts=0.1  seed=[90723]
  Band-Limited White Noise1 : simulink/Sources/Band-Limited White Noise  Cov=[0.001]  Ts=0.1  seed=[87324]
  Conversor A/D : Quantizer  QuantizationInterval=7.629e-5
  Conversor A/D1 : Quantizer  QuantizationInterval=0.00244
  ISA Atmosphere Model : aerolibatmos2/ISA Atmosphere Model  custom=on  g=9.80665  gamma=1.4  R=287.0531  L=0.0065  h_trop=11000  h_strat=20000  rho0=1.225  P0=101325  T0=288.15  h0=0
  Product : Product
  "Product  " : Product  Inputs=3
  Sum : Sum  Inputs=|++
  Temperature Conversion : aerolibconvert2/Temperature Conversion  IU=K  OU=C
  Voltage : Sum  Inputs=+++
  "b0 " : Fcn  Expr=(4.227e-1+1.513e-2*u)/(8.615e1+u)
  b1 : Constant  Value=0.0023
  "b2 " : Constant  Value=1.926e-6
  V : Outport
  b0 : Outport  Port=2
  wires:
  b1/1 -> Product/2
  h/1 -> ISA Atmosphere Model/1
  "b0 "/1 -> b0/1, Voltage/1
  Product/1 -> Voltage/2
  ISA Atmosphere Model/1 -> Temperature Conversion/1
  ISA Atmosphere Model/3 -> "Product  "/2, "Product  "/1, Product/1
  "Product  "/1 -> Voltage/3
  Voltage/1 -> Sum/1
  "b2 "/1 -> "Product  "/3
  Band-Limited White Noise/1 -> Sum/2
  Sum/1 -> Conversor A/D/1
  Conversor A/D/1 -> V/1
  Temperature Conversion/1 -> "  "/2
  "  "/1 -> Conversor A/D1/1
  Conversor A/D1/1 -> "b0 "/1
  Band-Limited White Noise1/1 -> "  "/1

== system fault_tolerant_controller/Model/Sensor Pressão Estática2 ==
  h : Inport
  "  " : Sum
  Band-Limited White Noise : simulink/Sources/Band-Limited White Noise  Cov=[25]  Ts=0.1  seed=[12987]
  Band-Limited White Noise1 : simulink/Sources/Band-Limited White Noise  Cov=[0.001]  Ts=0.1  seed=[79487]
  Conversor A/D : Quantizer  QuantizationInterval=7.629e-5
  Conversor A/D1 : Quantizer  QuantizationInterval=0.00244
  ISA Atmosphere Model : aerolibatmos2/ISA Atmosphere Model  custom=on  g=9.80665  gamma=1.4  R=287.0531  L=0.0065  h_trop=11000  h_strat=20000  rho0=1.225  P0=101325  T0=288.15  h0=0
  Product : Product
  "Product  " : Product  Inputs=3
  Sum : Sum  Inputs=|++
  Temperature Conversion : aerolibconvert2/Temperature Conversion  IU=K  OU=C
  Voltage : Sum  Inputs=+++
  "b0 " : Fcn  Expr=(4.227e-1+1.513e-2*u)/(8.615e1+u)
  b1 : Constant  Value=0.0023
  "b2 " : Constant  Value=1.926e-6
  V : Outport
  b0 : Outport  Port=2
  wires:
  b1/1 -> Product/2
  h/1 -> ISA Atmosphere Model/1
  "b0 "/1 -> b0/1, Voltage/1
  Product/1 -> Voltage/2
  ISA Atmosphere Model/1 -> Temperature Conversion/1
  ISA Atmosphere Model/3 -> "Product  "/2, "Product  "/1, Product/1
  "Product  "/1 -> Voltage/3
  Voltage/1 -> Sum/1
  "b2 "/1 -> "Product  "/3
  Band-Limited White Noise/1 -> Sum/2
  Sum/1 -> Conversor A/D/1
  Conversor A/D/1 -> V/1
  Temperature Conversion/1 -> "  "/2
  "  "/1 -> Conversor A/D1/1
  Conversor A/D1/1 -> "b0 "/1
  Band-Limited White Noise1/1 -> "  "/1

== system fault_tolerant_controller/Model/Sensor Pressão Estática3 ==
  h : Inport
  "  " : Sum
  Band-Limited White Noise : simulink/Sources/Band-Limited White Noise  Cov=[25]  Ts=0.1  seed=[88641]
  Band-Limited White Noise1 : simulink/Sources/Band-Limited White Noise  Cov=[0.001]  Ts=0.1  seed=[55298]
  Conversor A/D : Quantizer  QuantizationInterval=7.629e-5
  Conversor A/D1 : Quantizer  QuantizationInterval=0.00244
  ISA Atmosphere Model : aerolibatmos2/ISA Atmosphere Model  custom=on  g=9.80665  gamma=1.4  R=287.0531  L=0.0065  h_trop=11000  h_strat=20000  rho0=1.225  P0=101325  T0=288.15  h0=0
  Product : Product
  "Product  " : Product  Inputs=3
  Sum : Sum  Inputs=|++
  Temperature Conversion : aerolibconvert2/Temperature Conversion  IU=K  OU=C
  Voltage : Sum  Inputs=+++
  "b0 " : Fcn  Expr=(4.227e-1+1.513e-2*u)/(8.615e1+u)
  b1 : Constant  Value=0.0023
  "b2 " : Constant  Value=1.926e-6
  V : Outport
  b0 : Outport  Port=2
  wires:
  b1/1 -> Product/2
  h/1 -> ISA Atmosphere Model/1
  "b0 "/1 -> b0/1, Voltage/1
  Product/1 -> Voltage/2
  ISA Atmosphere Model/1 -> Temperature Conversion/1
  ISA Atmosphere Model/3 -> "Product  "/2, "Product  "/1, Product/1
  "Product  "/1 -> Voltage/3
  Voltage/1 -> Sum/1
  "b2 "/1 -> "Product  "/3
  Band-Limited White Noise/1 -> Sum/2
  Sum/1 -> Conversor A/D/1
  Conversor A/D/1 -> V/1
  Temperature Conversion/1 -> "  "/2
  "  "/1 -> Conversor A/D1/1
  Conversor A/D1/1 -> "b0 "/1
  Band-Limited White Noise1/1 -> "  "/1

== system fault_tolerant_controller/Model/Sensor Pressão Total ==
  airspeed : Inport
  h : Inport  Port=2
  "  " : Gain  Gain=0.5
  Band-Limited White Noise : simulink/Sources/Band-Limited White Noise  Cov=[1e-7]  Ts=0.1  seed=[14732]
  "Conversor A/D  " : Quantizer  QuantizationInterval=7.629e-5
  ISA Atmosphere Model : aerolibatmos2/ISA Atmosphere Model  custom=on  g=9.80665  gamma=1.4  R=287.0531  L=0.0065  h_trop=11000  h_strat=20000  rho0=1.225  P0=101325  T0=288.15  h0=0
  Pressão Dinâmica : Product  Inputs=3
  Pressão Total : Sum
  Sum6 : Sum  Inputs=|++
  "Voltage " : Fcn  Expr=u*(5/165125)
  V : Outport
  "h " : Outport  Port=2
  wires:
  airspeed/1 -> Pressão Dinâmica/2, Pressão Dinâmica/1
  h/1 -> "h "/1, ISA Atmosphere Model/1
  "Voltage "/1 -> Sum6/1
  ISA Atmosphere Model/4 -> "  "/1
  "  "/1 -> Pressão Dinâmica/3
  Band-Limited White Noise/1 -> Sum6/2
  Sum6/1 -> "Conversor A/D  "/1
  "Conversor A/D  "/1 -> V/1
  Pressão Dinâmica/1 -> Pressão Total/1
  Pressão Total/1 -> "Voltage "/1
  ISA Atmosphere Model/3 -> Pressão Total/2

== system fault_tolerant_controller/Model/Sensor Pressão Total1 ==
  airspeed : Inport
  h : Inport  Port=2
  "  " : Gain  Gain=0.5
  Band-Limited White Noise : simulink/Sources/Band-Limited White Noise  Cov=[1e-7]  Ts=0.1  seed=[11618]
  "Conversor A/D  " : Quantizer  QuantizationInterval=7.629e-5
  ISA Atmosphere Model : aerolibatmos2/ISA Atmosphere Model  custom=on  g=9.80665  gamma=1.4  R=287.0531  L=0.0065  h_trop=11000  h_strat=20000  rho0=1.225  P0=101325  T0=288.15  h0=0
  Pressão Dinâmica : Product  Inputs=3
  Pressão Total : Sum
  Sum6 : Sum  Inputs=|++
  "Voltage " : Fcn  Expr=u*(5/165125)
  V : Outport
  "h " : Outport  Port=2
  wires:
  airspeed/1 -> Pressão Dinâmica/2, Pressão Dinâmica/1
  h/1 -> "h "/1, ISA Atmosphere Model/1
  "Voltage "/1 -> Sum6/1
  ISA Atmosphere Model/4 -> "  "/1
  "  "/1 -> Pressão Dinâmica/3
  Band-Limited White Noise/1 -> Sum6/2
  Sum6/1 -> "Conversor A/D  "/1
  "Conversor A/D  "/1 -> V/1
  Pressão Dinâmica/1 -> Pressão Total/1
  Pressão Total/1 -> "Voltage "/1
  ISA Atmosphere Model/3 -> Pressão Total/2

== system fault_tolerant_controller/Model/Sensor Pressão Total2 ==
  airspeed : Inport
  h : Inport  Port=2
  "  " : Gain  Gain=0.5
  Band-Limited White Noise : simulink/Sources/Band-Limited White Noise  Cov=[1e-7]  Ts=0.1  seed=[99415]
  "Conversor A/D  " : Quantizer  QuantizationInterval=7.629e-5
  ISA Atmosphere Model : aerolibatmos2/ISA Atmosphere Model  custom=on  g=9.80665  gamma=1.4  R=287.0531  L=0.0065  h_trop=11000  h_strat=20000  rho0=1.225  P0=101325  T0=288.15  h0=0
  Pressão Dinâmica : Product  Inputs=3
  Pressão Total : Sum
  Sum6 : Sum  Inputs=|++
  "Voltage " : Fcn  Expr=u*(5/165125)
  V : Outport
  "h " : Outport  Port=2
  wires:
  airspeed/1 -> Pressão Dinâmica/2, Pressão Dinâmica/1
  h/1 -> "h "/1, ISA Atmosphere Model/1
  "Voltage "/1 -> Sum6/1
  ISA Atmosphere Model/4 -> "  "/1
  "  "/1 -> Pressão Dinâmica/3
  Band-Limited White Noise/1 -> Sum6/2
  Sum6/1 -> "Conversor A/D  "/1
  "Conversor A/D  "/1 -> V/1
  Pressão Dinâmica/1 -> Pressão Total/1
  Pressão Total/1 -> "Voltage "/1
  ISA Atmosphere Model/3 -> Pressão Total/2

== system fault_tolerant_controller/Model/Sensor Pressão Total3 ==
  airspeed : Inport
  h : Inport  Port=2
  "  " : Gain  Gain=0.5
  Band-Limited White Noise : simulink/Sources/Band-Limited White Noise  Cov=[1e-7]  Ts=0.1  seed=[43471]
  "Conversor A/D  " : Quantizer  QuantizationInterval=7.629e-5
  ISA Atmosphere Model : aerolibatmos2/ISA Atmosphere Model  custom=on  g=9.80665  gamma=1.4  R=287.0531  L=0.0065  h_trop=11000  h_strat=20000  rho0=1.225  P0=101325  T0=288.15  h0=0
  Pressão Dinâmica : Product  Inputs=3
  Pressão Total : Sum
  Sum6 : Sum  Inputs=|++
  "Voltage " : Fcn  Expr=u*(5/165125)
  V : Outport
  "h " : Outport  Port=2
  wires:
  airspeed/1 -> Pressão Dinâmica/2, Pressão Dinâmica/1
  h/1 -> "h "/1, ISA Atmosphere Model/1
  "Voltage "/1 -> Sum6/1
  ISA Atmosphere Model/4 -> "  "/1
  "  "/1 -> Pressão Dinâmica/3
  Band-Limited White Noise/1 -> Sum6/2
  Sum6/1 -> "Conversor A/D  "/1
  "Conversor A/D  "/1 -> V/1
  Pressão Dinâmica/1 -> Pressão Total/1
  Pressão Total/1 -> "Voltage "/1
  ISA Atmosphere Model/3 -> Pressão Total/2

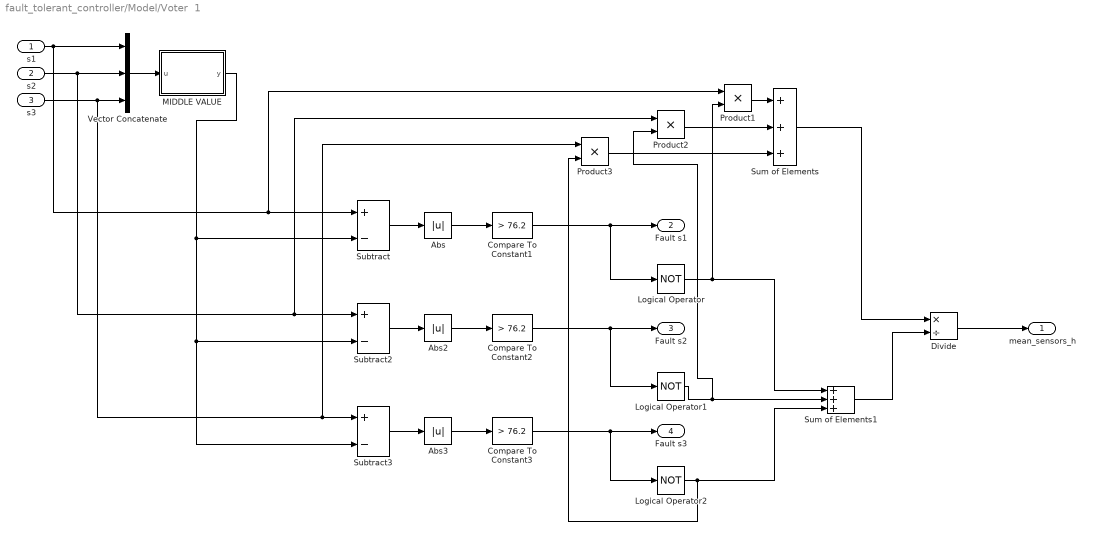
== system fault_tolerant_controller/Model/Voter  1 ==
  s1 : Inport
  s2 : Inport  Port=2
  s3 : Inport  Port=3
  Abs : Abs
  Abs2 : Abs
  Abs3 : Abs
  Compare To Constant1 : simulink/Logic and Bit Operations/Compare To Constant  relop=>  const=76.2  OutDataTypeStr=boolean
  Compare To Constant2 : simulink/Logic and Bit Operations/Compare To Constant  relop=>  const=76.2  OutDataTypeStr=boolean
  Compare To Constant3 : simulink/Logic and Bit Operations/Compare To Constant  relop=>  const=76.2  OutDataTypeStr=boolean
  Divide : Product  Inputs=*/
  Logical Operator : Logic  Operator=NOT  AllPortsSameDT=off  OutDataTypeStr=boolean
  Logical Operator1 : Logic  Operator=NOT  AllPortsSameDT=off  OutDataTypeStr=boolean
  Logical Operator2 : Logic  Operator=NOT  AllPortsSameDT=off  OutDataTypeStr=boolean
  "MIDDLE VALUE " : MATLAB Function  TreatAsAtomicUnit=on
  Product1 : Product
  Product2 : Product
  Product3 : Product
  Subtract : Sum  Inputs=+-
  Subtract2 : Sum  Inputs=+-
  Subtract3 : Sum  Inputs=+-
  Sum of Elements : Sum  Inputs=+++
  Sum of Elements1 : Sum  Inputs=+++
  Vector Concatenate : Concatenate  NumInputs=3
  " mean_sensors_h" : Outport
  "Fault s1  " : Outport  Port=2
  "Fault s2  " : Outport  Port=3
  "Fault s3  " : Outport  Port=4
  wires:
  Vector Concatenate/1 -> "MIDDLE VALUE "/1(u)
  Subtract3/1 -> Abs3/1
  Subtract/1 -> Abs/1
  s3/1 -> Product3/1, Subtract3/1, Vector Concatenate/3
  Subtract2/1 -> Abs2/1
  "MIDDLE VALUE "/1(y) -> Subtract/2, Subtract3/2, Subtract2/2
  Sum of Elements/1 -> Divide/1
  Sum of Elements1/1 -> Divide/2
  Divide/1 -> " mean_sensors_h"/1
  Abs/1 -> Compare To Constant1/1
  Compare To Constant1/1 -> Logical Operator/1, "Fault s1  "/1
  Compare To Constant2/1 -> Logical Operator1/1, "Fault s2  "/1
  Abs2/1 -> Compare To Constant2/1
  Abs3/1 -> Compare To Constant3/1
  Compare To Constant3/1 -> Logical Operator2/1, "Fault s3  "/1
  Logical Operator/1 -> Product1/2, Sum of Elements1/1
  Logical Operator1/1 -> Sum of Elements1/2, Product2/2
  Logical Operator2/1 -> Sum of Elements1/3, Product3/2
  s1/1 -> Product1/1, Subtract/1, Vector Concatenate/1
  s2/1 -> Product2/1, Subtract2/1, Vector Concatenate/2
  Product2/1 -> Sum of Elements/2
  Product3/1 -> Sum of Elements/3
  Product1/1 -> Sum of Elements/1
